simulink model "model2bis"  (R2015a)
settings: Solver=ode4  StartTime=0.0  StopTime=20.0  FixedStep=0.01  RelTol=1e-3
settings Model: Creator=jleny  LastModifiedBy=jleny

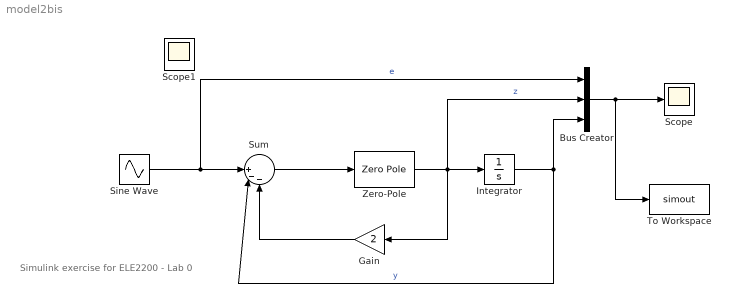
== system model2bis ==
  note: Simulink exercise for ELE2200 - Lab 0
  Bus Creator : BusCreator  Inputs=3
  Gain : Gain  Gain=2
  Integrator : Integrator
  Scope : Scope
      settings: ShowLegends=on
  Sine Wave : Sin  Amplitude=0.1  Bias=1  Frequency=5  SampleTime=0
  Sum : Sum  Inputs=||+--
  To Workspace : ToWorkspace  VariableName=simout  SaveFormat=Timeseries  SampleTime=-1
  Zero-Pole : ZeroPole  Zeros=[-5]  Poles=[0 -10]  Gain=[2]
  Scope1 : Scope
  wires:
  Sine Wave/1 -> Bus Creator/1, Sum/1  "e"
  Zero-Pole/1 -> Bus Creator/2, Gain/1, Integrator/1  "z"
  Gain/1 -> Sum/3
  Sum/1 -> Zero-Pole/1
  Integrator/1 -> Bus Creator/3, Sum/2  "y"
  Bus Creator/1 -> Scope/1, To Workspace/1
